simulink model "Two_Zone_MVDC_PSolver_Thermal"  (R2025b)
settings: Solver=FixedStepDiscrete  StartTime=0.0  StopTime=30  FixedStep=TsELEC  RelTol=1e-3  EnableMultiTasking=on
InitFcn:
  | TsELEC = 25e-6;
  | Ts = 25e-6;
  | TsTHERMAL = 1e-3;
  | TsCont = TsELEC;
  | Rsnub = 1e4;
undefined symbols (not defined in the file or in its folder): DiscIntNeverNeededParam, ee_sli_rtmsupport, GABDA, GABDB, GBBDA, GBBDB, gcbh, GPMMA, GPPMB, GPPMC, SADA, SADB, SADC, SADD, SBDA, SBDB, SBDC, SCDA, SCDB, SCDC, SCDD, SDDA, SDDB, SDDC, SDDD, SDDE
libraries: fl_lib x182, nesl_utility x93, ee_lib x50, SimscapeFluids_lib x4, simulink x3, slpidlib x3, eeSmAC1C x2, eePowerMeasurement x2, mcbeeMathTransformLib x2, eeTransforms x1
(part 3 of 5)

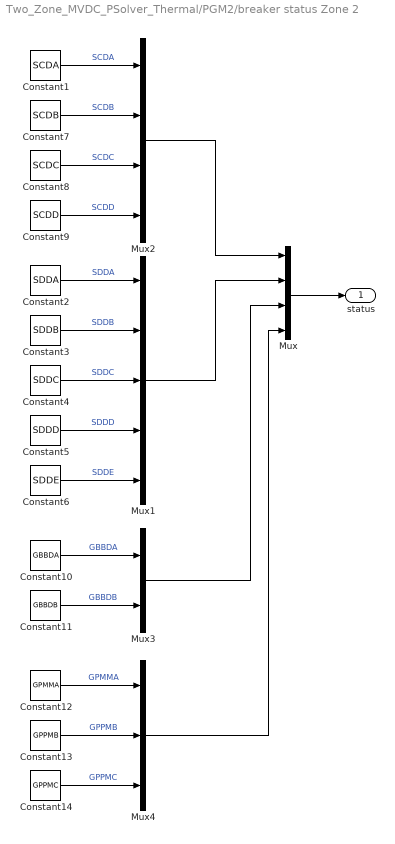
== system Two_Zone_MVDC_PSolver_Thermal/PGM2/breaker status Zone 2 ==
  Constant1 : Constant  Value=SCDA  SampleTime=Ts
  Constant10 : Constant  Value=GBBDA  SampleTime=Ts
  Constant11 : Constant  Value=GBBDB  SampleTime=Ts
  Constant12 : Constant  Value=GPMMA  SampleTime=Ts
  Constant13 : Constant  Value=GPPMB  SampleTime=Ts
  Constant14 : Constant  Value=GPPMC  SampleTime=Ts
  Constant2 : Constant  Value=SDDA  SampleTime=Ts
  Constant3 : Constant  Value=SDDB  SampleTime=Ts
  Constant4 : Constant  Value=SDDC  VectorParams1D=off  SampleTime=Ts
  Constant5 : Constant  Value=SDDD  SampleTime=Ts
  Constant6 : Constant  Value=SDDE  SampleTime=Ts
  Constant7 : Constant  Value=SCDB  SampleTime=Ts
  Constant8 : Constant  Value=SCDC  SampleTime=Ts
  Constant9 : Constant  Value=SCDD  SampleTime=Ts
  Mux : Mux  Inputs=[4 5 2 3]
  Mux1 : Mux  Inputs=5
  Mux2 : Mux
  Mux3 : Mux  Inputs=2
  Mux4 : Mux  Inputs=3
  status : Outport  VectorParamsAs1DForOutWhenUnconnected=off
  wires:
  Mux/1 -> status/1
  Constant9/1 -> Mux2/4  "SCDD"
  Constant8/1 -> Mux2/3  "SCDC"
  Constant7/1 -> Mux2/2  "SCDB"
  Constant1/1 -> Mux2/1  "SCDA"
  Constant6/1 -> Mux1/5  "SDDE"
  Constant4/1 -> Mux1/3  "SDDC"
  Constant3/1 -> Mux1/2  "SDDB"
  Constant2/1 -> Mux1/1  "SDDA"
  Constant5/1 -> Mux1/4  "SDDD"
  Constant10/1 -> Mux3/1  "GBBDA"
  Constant11/1 -> Mux3/2  "GBBDB"
  Constant12/1 -> Mux4/1  "GPMMA"
  Constant13/1 -> Mux4/2  "GPPMB"
  Constant14/1 -> Mux4/3  "GPPMC"
  Mux2/1 -> Mux/1
  Mux1/1 -> Mux/2
  Mux3/1 -> Mux/3
  Mux4/1 -> Mux/4

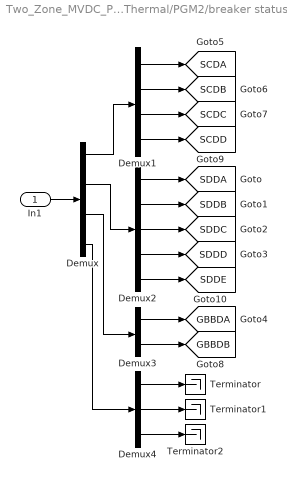
== system Two_Zone_MVDC_PSolver_Thermal/PGM2/breaker status1 ==
  In1 : Inport
  Demux : Demux  Outputs=[4 5 2 3]
  Demux1 : Demux
  Demux2 : Demux  Outputs=5
  Demux3 : Demux  Outputs=2
  Demux4 : Demux  Outputs=3
  Terminator : Terminator
  Terminator1 : Terminator
  Terminator2 : Terminator
  tag scope: GBBDA=global, GBBDB=global, SCDA=global, SCDB=global, SCDC=global, SCDD=global, SDDA=global, SDDB=global, SDDC=global, SDDD=global, SDDE=global
  wires:
  Demux/4 -> Demux4/1
  Demux4/3 -> Terminator2/1
  Demux4/2 -> Terminator1/1
  Demux4/1 -> Terminator/1
  Demux/3 -> Demux3/1
  Demux3/2 -> [GBBDB]
  Demux3/1 -> [GBBDA]
  Demux/2 -> Demux2/1
  Demux/1 -> Demux1/1
  Demux2/5 -> [SDDE]
  Demux1/4 -> [SCDD]
  Demux1/3 -> [SCDC]
  Demux1/2 -> [SCDB]
  Demux1/1 -> [SCDA]
  In1/1 -> Demux/1
  Demux2/4 -> [SDDD]
  Demux2/3 -> [SDDC]
  Demux2/1 -> [SDDA]
  Demux2/2 -> [SDDB]

== system Two_Zone_MVDC_PSolver_Thermal/PMM/Control ==
  Selector : Selector  InputPortWidth=2  IndexOptions=Index vector (dialog)  Indices=2  OutputSizes=1
  Selector1 : Selector  InputPortWidth=2  IndexOptions=Index vector (dialog)  Indices=1  OutputSizes=1
  Speed Control : Subsystem
  Torque Control : Subsystem
  Unit Delay1 : UnitDelay  SampleTime=Ts  HasFrameUpgradeWarning=on
  duty_cycle : Outport
  wires:
  Speed Control/1(IdqRef_PU) -> Torque Control/1(Idq_ref_PU)
  Selector1/1 -> Torque Control/3(Pos_Sim)
  Torque Control/1(Vabc_out_PU) -> Unit Delay1/1
  [Iab_meas1] -> Torque Control/2(Iab_Sim)
  Selector/1 -> Speed Control/2(Speed_Meas_PU)
  [pos_speed_1] -> Selector1/1, Selector/1
  [Nref1] -> Speed Control/1(Speed_Ref_PU)
  Unit Delay1/1 -> duty_cycle/1

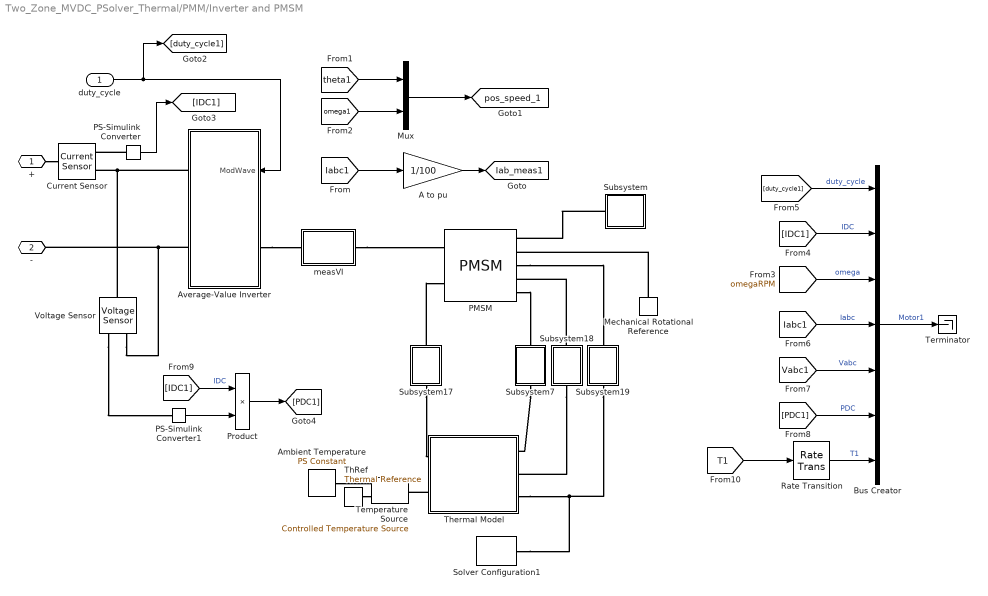
== system Two_Zone_MVDC_PSolver_Thermal/PMM/Inverter and PMSM ==
  duty_cycle : Inport
  A to pu : Gain  Gain=1/100
  Ambient Temperature : fl_lib/Physical Signals/Sources/PS Constant  constant=300
  Average-Value Inverter : Subsystem
  Bus Creator : BusCreator  Inputs=7
  Current Sensor : fl_lib/Electrical/Electrical Sensors/Current Sensor
  Mechanical Rotational Reference : fl_lib/Mechanical/Rotational Elements/Mechanical Rotational Reference
  Mux : Mux  Inputs=2
  PMSM : ee_lib/Electromechanical/Permanent Magnet/PMSM  port_option=ee.enum.threePhasePort.composite  winding_type=ee.enum.statorconnection.wye  machine_param=ee.enum.pmsm.parameterization.constant  nPolePairs=1  pmflux_param=ee.enum.pmflux.fluxlinkage  pm_flux_linkage=3.15*4 Wb  torque_constant=0.18 N*m/A  back_emf_constant=0.18 V/(rad/s)  stator_param=ee.enum.statorparam.LdLqL0  Ld=0.002 H  Lq=0.002 H  idVec=[-200, 0, 200] A  iqVec=[-200, 0, 200] A  LdMatrix=0.0002 * ones(3, 3) H  LqMatrix=0.0002 * ones(3, 3) H  PmMatrix=0.1 * ones(3, 3) Wb  ktMatrix=0.18 * ones(3, 3) N*m/A  keMatrix=0.18 * ones(3, 3) V/(rad/s)  L0=0 H  Ls=0.0002 H  Lm=-0.00002 H  Ms=0.00002 H  Rs=0.01 Ohm  zero_sequence=ee.enum.park.zerosequence.exclude  axes_param=ee.enum.rotorangle.daxis  loss_param=ee.enum.ironloss.none  losses_oc=[0, 0, 0] W  losses_sc=[0, 0, 0] W  f_losses=60 Hz  Isc_losses=95 A  J=2 kg*m^2  lam=1 N*m/(rad/s)  i_d_specify=off  i_d_priority=None  i_d=0 A  i_d_nominal_specify=off  i_d_nominal_value=1  i_d_nominal_unit=A  i_q_specify=off  i_q_priority=None  i_q=0 A  i_q_nominal_specify=off  i_q_nominal_value=1  i_q_nominal_unit=A  torque_specify=off  torque_priority=None  torque=0 N*m  torque_nominal_specify=off  torque_nominal_value=1  torque_nominal_unit=N*m  angular_velocity_specify=off  angular_velocity_priority=High  angular_velocity=0 rpm  angular_velocity_nominal_specify=off  angular_velocity_nominal_value=1  angular_velocity_nominal_unit=rpm  angular_position_specify=off  angular_position_priority=High  angular_position=0 deg  angular_position_nominal_specify=off  angular_position_nominal_value=1  angular_position_nominal_unit=deg  alpha=1e-6 1/K  alpha_flux=-0.001 1/K  Tmeas=298.15 K  stator_thermal_mass=1000 J/K  rotor_thermal_mass=2000 J/K  Rm_percent_rotor=90  Rd_percent_rotor=30  temperatureA_specify=off  temperatureA_priority=High  temperatureA=25 degC  temperatureA_nominal_specify=off  temperatureA_nominal_value=1  temperatureA_nominal_unit=degC  temperatureB_specify=off  temperatureB_priority=High  temperatureB=25 degC  temperatureB_nominal_specify=off  temperatureB_nominal_value=1  temperatureB_nominal_unit=degC  temperatureC_specify=off  temperatureC_priority=High  temperatureC=25 degC  temperatureC_nominal_specify=off  temperatureC_nominal_value=1  temperatureC_nominal_unit=degC  temperatureR_specify=off  temperatureR_priority=High  temperatureR=25 degC  temperatureR_nominal_specify=off  temperatureR_nominal_value=1  temperatureR_nominal_unit=degC
      settings: InternalSimscapePortConfiguration="{\"Bottom\":[],\"Left\":[{\"id\":\"N\",\"label\":\"~\",\"type\":\"foundation.electrical.three_phase\"},{\"id\":\"HR\",\"label\":\"HR\",\"type\":\"foundation.thermal.thermal\"}],\"Right\":[{\"id\":\"R\",\"label\":\"R\",\"type\":\"foundation.mechanical.rotational.rotational\"},{\"id\":\"C\",\"label\":\"C\",\"type\":\"foundation.mechanical.rotational.rotational\"},{\"id\":\"HA\",\"label\":\"HA\",\"type\":\"foundation.thermal.thermal\"},{\"id\":\"HB\",\"label\":\"HB\",\"type\":\"foundation.thermal.thermal\"},{\"id\":\"HC\",\"label\":\"HC\",\"type\":\"foundation.thermal.thermal\"}],\"Top\":[]}"
  PS-Simulink Converter : nesl_utility/PS-Simulink Converter  PhysicalDomain=network_engine_domain  SubClassName=ps_output  LeftPortType=input  RightPortType=output  PseudoPeriodic=off  Frequencies=[]  VectorFormat=1-D array  Unit=inherit  AffineConversion=off
  PS-Simulink Converter1 : nesl_utility/PS-Simulink Converter  PhysicalDomain=network_engine_domain  SubClassName=ps_output  LeftPortType=input  RightPortType=output  PseudoPeriodic=off  Frequencies=[]  VectorFormat=1-D array  Unit=inherit  AffineConversion=off
  Product : Product
  Rate Transition : RateTransition
  Solver Configuration1 : nesl_utility/Solver Configuration  PhysicalDomain=network_engine_domain  SubClassName=solver  LeftPortType=input  RightPortType=generic  Tones=[]  Harmonics=[]  SimulateNoise=off  Profile=off  UseLocalSampling=off  EnableSwitchedLinearOptims=on  FrequencyDomain=off  UseCCode=off  RelTol=0.001  AbsTol=1e-06  MinStep=1e-09  ToWorkspace=off  RevertToSquareIcSolve=off  NumHomotopyIterations=100  PhasorMode=off  PhasorModeNumHarmonics=1  ConsistencySolver=NEWTON_FTOL  IndexReductionMethod=DerivativeReplacement  DoDC=off  ResidualTolerance=1e-9  ConsistencyTolSource=GLOBAL  ConsistencyAbsTol=0.001  ConsistencyRelTol=0.001  ConsistencyTolFactor=0.001  UseLocalSolver=on  LocalSolverChoice=NE_BACKWARD_EULER_ADVANCER  ResolveIndetEquations=on  FunctionEvalNumThread=1  LocalSolverSampleTime=TsTHERMAL  DoFixedCost=on  MaxNonlinIter=1  MaxModeIter=2  ComputeImpulses=off  ImpulseIterations=2  LinearAlgebra=Full  LinearAlgebraNumThread=0  EquationFormulation=NE_TIME_EF  DelaysMemoryBudget=1024  AutomaticFiltering=on  FilteringTimeConstant=0.001  PartitionStorageMethod=AS_NEEDED  PartitionMemoryBudget=1024  PartitionMethod=FAST  MultibodyUseLocalSolver=off  MultibodyLocalSolverChoice=ODE1  MultibodyLocalSolverSampleTime=0.001
  Subsystem : Subsystem
  Subsystem17 : Subsystem
  Subsystem18 : Subsystem
  Subsystem19 : Subsystem
  Subsystem7 : Subsystem
  Temperature Source : fl_lib/Thermal/Thermal Sources/Controlled Temperature Source
  Terminator : Terminator
  ThRef : fl_lib/Thermal/Thermal Elements/Thermal Reference
  Thermal Model : Subsystem  Tag=PublishSubsystem
  Voltage Sensor : fl_lib/Electrical/Electrical Sensors/Voltage Sensor
  measVI : Subsystem
  + : PMIOPort  Side=Left
  - : PMIOPort  Port=2  Side=Left
  tag scope: Iab_meas1=global, pos_speed_1=global
  wires:
  [Vabc1] -> Bus Creator/5  "Vabc"
  [Iabc1] -> Bus Creator/4  "Iabc"
  Bus Creator/1 -> Terminator/1  "Motor1"
  [omegaRPM] -> Bus Creator/3  "omega"
  [IDC1] -> Bus Creator/2  "IDC"
  [duty_cycle1] -> Bus Creator/1  "duty_cycle"
  PS-Simulink Converter/1 -> [IDC1]
  Mux/1 -> [pos_speed_1]
  [omega1] -> Mux/2
  [theta1] -> Mux/1
  [Iabc1] -> A to pu/1
  A to pu/1 -> [Iab_meas1]
  PS-Simulink Converter1/1 -> Product/2
  Product/1 -> [PDC1]
  [PDC1] -> Bus Creator/6  "PDC"
  [IDC1] -> Product/1  "IDC"
  duty_cycle/1 -> [duty_cycle1], Average-Value Inverter/1(ModWave)
  [T1] -> Rate Transition/1
  Rate Transition/1 -> Bus Creator/7  "T1"
  connections:
  Average-Value Inverter/RConn2 -- Voltage Sensor/RConn2 -- -/RConn1
  +/RConn1 -- Current Sensor/LConn1
  PS-Simulink Converter/LConn1 -- Current Sensor/RConn1
  Average-Value Inverter/RConn1 -- Voltage Sensor/LConn1 -- Current Sensor/RConn2
  measVI/RConn1 -- PMSM/LConn1
  Average-Value Inverter/LConn1 -- measVI/LConn1
  Subsystem/RConn1 -- PMSM/RConn1
  Mechanical Rotational Reference/LConn1 -- PMSM/RConn2
  Voltage Sensor/RConn1 -- PS-Simulink Converter1/LConn1
  Subsystem19/LConn1 -- Solver Configuration1/RConn1 -- Thermal Model/RConn3
  Subsystem7/LConn1 -- Thermal Model/RConn1
  Subsystem18/LConn1 -- Thermal Model/RConn2
  Subsystem17/LConn1 -- Thermal Model/LConn1
  ThRef/LConn1 -- Temperature Source/RConn2
  Thermal Model/LConn2 -- Temperature Source/LConn1
  Ambient Temperature/RConn1 -- Temperature Source/RConn1
  Subsystem17/RConn1 -- PMSM/LConn2
  PMSM/RConn3 -- Subsystem19/RConn1
  Subsystem18/RConn1 -- PMSM/RConn4
  PMSM/RConn5 -- Subsystem7/RConn1

== system Two_Zone_MVDC_PSolver_Thermal/PMM/Speed Reference ==
  LPF : Subsystem
  Power Reference : simulink/Sources/Repeating Sequence Interpolated  OutValues=[0 0 0.5 0.5 -0.5 -0.5]  TimeValues=[0 5 10 15 25 100]  LookUpMeth=Interpolation-Use End Values  tsamp=TsELEC  OutMin=[]  OutMax=[]  OutDataTypeStr=double  OutputDataTypeScalingMode=double  OutDataType=fixdt(0,8)  OutScaling=2^-10
  tag scope: Nref1=global
  wires:
  LPF/1(y) -> [Nref1]
  Power Reference/1 -> LPF/1(u)

== system Two_Zone_MVDC_PSolver_Thermal/PGM1/Gas turbine/ AC1C ==
  Constant1 : Constant  Value=0  SampleTime=TsCont
  Constant2 : Constant  Value=0  SampleTime=TsCont
  PS-Simulink Converter : nesl_utility/PS-Simulink Converter  PhysicalDomain=network_engine_domain  SubClassName=ps_output  LeftPortType=input  RightPortType=output  PseudoPeriodic=off  Frequencies=[]  VectorFormat=1-D array  Unit=inherit  AffineConversion=off
  PS-Simulink Converter1 : nesl_utility/PS-Simulink Converter  PhysicalDomain=network_engine_domain  SubClassName=ps_output  LeftPortType=input  RightPortType=output  PseudoPeriodic=off  Frequencies=[]  VectorFormat=1-D array  Unit=inherit  AffineConversion=off
  Rate Transition : RateTransition  OutPortSampleTime=TsELEC
  Rate Transition1 : RateTransition  OutPortSampleTime=TsCont
  Rate Transition2 : RateTransition  OutPortSampleTime=TsCont
  Repeating Sequence Interpolated2 : simulink/Sources/Repeating Sequence Interpolated  OutValues=[1 1 1]  TimeValues=[0 5 1000]  LookUpMeth=Interpolation-Use End Values  tsamp=TsCont  OutMin=[]  OutMax=[]  OutDataTypeStr=double  OutputDataTypeScalingMode=double  OutDataType=fixdt(0,8)  OutScaling=2^-10
  SM AC1C : eeSmAC1C/SM AC1C  E_FD0=1  Ts=TsCont  R_C=0  X_C=0  T_R=0  K_A=80  T_A=0.2  T_B=0  T_C=0  K_F=0.03  T_F=1.49  V_Amax=14.5  V_Amin=-14.5  E_FEmax=6.03  E_FEmin=-5.43  oelInputLocation=Unused  uelInputLocation=Unused  sclInputLocation=Unused  K_E=1  T_E=0.8  K_C=0.2  K_D=0.38  E_1=4.18  S_E_E1=0.1  E_2=3.14  S_E_E2=0.03  V_FEmax=99  V_Emin=0
      settings: LibrarySourceBlock=ee_sl_lib/SM Control/SM AC1C
  Simulink-PS Converter : nesl_utility/Simulink-PS Converter  PhysicalDomain=network_engine_domain  SubClassName=ps_input  LeftPortType=input  RightPortType=output  PseudoPeriodic=off  Frequencies=[]  NoiseDistribution=none  NoiseParameters=[]  Unit=1  AffineConversion=off  FilteringAndDerivatives=provide  SimscapeFilterOrder=1  InputFilterTimeConstant=0.001  UdotUserProvided=0
  Synchronous Machine Field Circuit (pu) : ee_lib/Electromechanical/Synchronous/Synchronous Machine Field Circuit  unit_option=ee.enum.unit.pu  SRated=36e6 V*A  FRated=60 Hz  fieldCircuitParameterization_option=ee.enum.sm.fieldparameterization.current  baseEfd=92.95 V  baseIfd=200 A  parameterization_option=ee.enum.sm.parameterization.standard  Ladu=1.66  Rfd=0.0006  Xl=0.15  Xd=1.81  Xdd=0.3  Xddd=0.23  d_option=ee.enum.circuit.open  Td0d=8 s  Tdd=1.3260 s  Td0dd=0.03 s  Tddd=0.0230 s
      settings: LogSimulationData=on  InternalSimscapePortConfiguration="{\"Bottom\":[],\"Left\":[{\"id\":\"Efd_pu\",\"label\":\"Efd_pu\",\"type\":\"input\"},{\"id\":\"Ifd_pu\",\"label\":\"Ifd_pu\",\"type\":\"output\"}],\"Right\":[{\"id\":\"fd_p\",\"label\":\"fd+\",\"type\":\"foundation.electrical.electrical\"},{\"id\":\"fd_n\",\"label\":\"fd-\",\"type\":\"foundation.electrical.electrical\"}],\"Top\":[]}"
  Terminal Voltage Measurement : ee_lib/Electromechanical/Synchronous/Synchronous Machine Measurement  output_idx=14
      settings: LogSimulationData=on  InternalSimscapePortConfiguration="{\"Bottom\":[],\"Left\":[{\"id\":\"pu_input\",\"label\":\"pu\",\"type\":\"input\"}],\"Right\":[{\"id\":\"pu_output\",\"label\":\"o\",\"type\":\"output\"}],\"Top\":[]}"
  Unit Delay : UnitDelay  InitialCondition=1.37673  SampleTime=-1  HasFrameUpgradeWarning=on
  pu : PMIOPort  Side=Left
  fd+ : PMIOPort  Port=2  Side=Right
  fd- : PMIOPort  Port=3  Side=Right
  wires:
  PS-Simulink Converter1/1 -> Unit Delay/1
  PS-Simulink Converter/1 -> Rate Transition1/1  "Vt1"
  Unit Delay/1 -> Rate Transition2/1  "Ifd1"
  Rate Transition/1 -> Simulink-PS Converter/1
  Repeating Sequence Interpolated2/1 -> SM AC1C/1
  Constant1/1 -> SM AC1C/2
  Rate Transition2/1 -> SM AC1C/10
  Rate Transition1/1 -> SM AC1C/3
  Constant2/1 -> SM AC1C/8, SM AC1C/7, SM AC1C/6, SM AC1C/5, SM AC1C/4, SM AC1C/9
  SM AC1C/1 -> Rate Transition/1
  connections:
  fd-/RConn1 -- Synchronous Machine Field Circuit (pu)/RConn2
  Synchronous Machine Field Circuit (pu)/RConn1 -- fd+/RConn1
  PS-Simulink Converter1/LConn1 -- Synchronous Machine Field Circuit (pu)/LConn2
  Simulink-PS Converter/RConn1 -- Synchronous Machine Field Circuit (pu)/LConn1
  pu/RConn1 -- Terminal Voltage Measurement/LConn1
  PS-Simulink Converter/LConn1 -- Terminal Voltage Measurement/RConn1

== system Two_Zone_MVDC_PSolver_Thermal/PGM1/Gas turbine/Turbine and governor  ==
  Gas Turbine : Subsystem
  Governor : Subsystem
  Ideal Torque Source : fl_lib/Mechanical/Mechanical Sources/Ideal Torque Source
  Mechanical Rotational Reference : fl_lib/Mechanical/Rotational Elements/Mechanical Rotational Reference
  scale by base_torque : fl_lib/Physical Signals/Functions/PS Gain  gain=base_torque N*m/s
  R : PMIOPort  Side=Right
  C : PMIOPort  Port=2  Side=Right
  pu : PMIOPort  Port=3  Side=Left
  connections:
  Gas Turbine/RConn1 -- scale by base_torque/LConn1
  scale by base_torque/RConn1 -- Ideal Torque Source/RConn1
  pu/RConn1 -- Governor/LConn1
  Governor/RConn1 -- Gas Turbine/LConn1
  Ideal Torque Source/LConn1 -- R/RConn1
  Mechanical Rotational Reference/LConn1 -- Ideal Torque Source/RConn2 -- C/RConn1

== system Two_Zone_MVDC_PSolver_Thermal/PGM2/Gas turbine/ AC1C ==
  Constant1 : Constant  Value=0  SampleTime=TsCont
  Constant2 : Constant  Value=0  SampleTime=TsCont
  PS-Simulink Converter : nesl_utility/PS-Simulink Converter  PhysicalDomain=network_engine_domain  SubClassName=ps_output  LeftPortType=input  RightPortType=output  PseudoPeriodic=off  Frequencies=[]  VectorFormat=1-D array  Unit=inherit  AffineConversion=off
  PS-Simulink Converter1 : nesl_utility/PS-Simulink Converter  PhysicalDomain=network_engine_domain  SubClassName=ps_output  LeftPortType=input  RightPortType=output  PseudoPeriodic=off  Frequencies=[]  VectorFormat=1-D array  Unit=inherit  AffineConversion=off
  Rate Transition : RateTransition  OutPortSampleTime=TsELEC
  Rate Transition1 : RateTransition  OutPortSampleTime=TsCont
  Rate Transition2 : RateTransition  OutPortSampleTime=TsCont
  Repeating Sequence Interpolated2 : simulink/Sources/Repeating Sequence Interpolated  OutValues=[1 1 1]  TimeValues=[0 5 1000]  LookUpMeth=Interpolation-Use End Values  tsamp=TsCont  OutMin=[]  OutMax=[]  OutDataTypeStr=double  OutputDataTypeScalingMode=double  OutDataType=fixdt(0,8)  OutScaling=2^-10
  SM AC1C : eeSmAC1C/SM AC1C  E_FD0=1  Ts=TsCont  R_C=0  X_C=0  T_R=0  K_A=80  T_A=0.2  T_B=0  T_C=0  K_F=0.03  T_F=1.49  V_Amax=14.5  V_Amin=-14.5  E_FEmax=6.03  E_FEmin=-5.43  oelInputLocation=Unused  uelInputLocation=Unused  sclInputLocation=Unused  K_E=1  T_E=0.8  K_C=0.2  K_D=0.38  E_1=4.18  S_E_E1=0.1  E_2=3.14  S_E_E2=0.03  V_FEmax=99  V_Emin=0
      settings: LibrarySourceBlock=ee_sl_lib/SM Control/SM AC1C
  Simulink-PS Converter : nesl_utility/Simulink-PS Converter  PhysicalDomain=network_engine_domain  SubClassName=ps_input  LeftPortType=input  RightPortType=output  PseudoPeriodic=off  Frequencies=[]  NoiseDistribution=none  NoiseParameters=[]  Unit=1  AffineConversion=off  FilteringAndDerivatives=provide  SimscapeFilterOrder=1  InputFilterTimeConstant=0.001  UdotUserProvided=0
  Synchronous Machine Field Circuit (pu) : ee_lib/Electromechanical/Synchronous/Synchronous Machine Field Circuit  unit_option=ee.enum.unit.pu  SRated=36e6 V*A  FRated=60 Hz  fieldCircuitParameterization_option=ee.enum.sm.fieldparameterization.current  baseEfd=92.95 V  baseIfd=200 A  parameterization_option=ee.enum.sm.parameterization.standard  Ladu=1.66  Rfd=0.0006  Xl=0.15  Xd=1.81  Xdd=0.3  Xddd=0.23  d_option=ee.enum.circuit.open  Td0d=8 s  Tdd=1.3260 s  Td0dd=0.03 s  Tddd=0.0230 s
      settings: LogSimulationData=on  InternalSimscapePortConfiguration="{\"Bottom\":[],\"Left\":[{\"id\":\"Efd_pu\",\"label\":\"Efd_pu\",\"type\":\"input\"},{\"id\":\"Ifd_pu\",\"label\":\"Ifd_pu\",\"type\":\"output\"}],\"Right\":[{\"id\":\"fd_p\",\"label\":\"fd+\",\"type\":\"foundation.electrical.electrical\"},{\"id\":\"fd_n\",\"label\":\"fd-\",\"type\":\"foundation.electrical.electrical\"}],\"Top\":[]}"
  Terminal Voltage Measurement : ee_lib/Electromechanical/Synchronous/Synchronous Machine Measurement  output_idx=14
      settings: LogSimulationData=on  InternalSimscapePortConfiguration="{\"Bottom\":[],\"Left\":[{\"id\":\"pu_input\",\"label\":\"pu\",\"type\":\"input\"}],\"Right\":[{\"id\":\"pu_output\",\"label\":\"o\",\"type\":\"output\"}],\"Top\":[]}"
  Unit Delay : UnitDelay  InitialCondition=1.37673  SampleTime=-1  HasFrameUpgradeWarning=on
  pu : PMIOPort  Side=Left
  fd+ : PMIOPort  Port=2  Side=Right
  fd- : PMIOPort  Port=3  Side=Right
  wires:
  PS-Simulink Converter1/1 -> Unit Delay/1
  PS-Simulink Converter/1 -> Rate Transition1/1  "Vt2"
  Unit Delay/1 -> Rate Transition2/1  "Ifd2"
  Rate Transition/1 -> Simulink-PS Converter/1
  Repeating Sequence Interpolated2/1 -> SM AC1C/1
  Constant1/1 -> SM AC1C/2
  Rate Transition2/1 -> SM AC1C/10
  Rate Transition1/1 -> SM AC1C/3
  Constant2/1 -> SM AC1C/8, SM AC1C/7, SM AC1C/6, SM AC1C/5, SM AC1C/4, SM AC1C/9
  SM AC1C/1 -> Rate Transition/1
  connections:
  fd-/RConn1 -- Synchronous Machine Field Circuit (pu)/RConn2
  Synchronous Machine Field Circuit (pu)/RConn1 -- fd+/RConn1
  PS-Simulink Converter1/LConn1 -- Synchronous Machine Field Circuit (pu)/LConn2
  Simulink-PS Converter/RConn1 -- Synchronous Machine Field Circuit (pu)/LConn1
  pu/RConn1 -- Terminal Voltage Measurement/LConn1
  PS-Simulink Converter/LConn1 -- Terminal Voltage Measurement/RConn1

== system Two_Zone_MVDC_PSolver_Thermal/PGM2/Gas turbine/Turbine and governor  ==
  Gas Turbine : Subsystem
  Governor : Subsystem
  Ideal Torque Source : fl_lib/Mechanical/Mechanical Sources/Ideal Torque Source
  Mechanical Rotational Reference : fl_lib/Mechanical/Rotational Elements/Mechanical Rotational Reference
  scale by base_torque : fl_lib/Physical Signals/Functions/PS Gain  gain=base_torque N*m/s
  R : PMIOPort  Side=Right
  C : PMIOPort  Port=2  Side=Right
  pu : PMIOPort  Port=3  Side=Left
  connections:
  Gas Turbine/RConn1 -- scale by base_torque/LConn1
  scale by base_torque/RConn1 -- Ideal Torque Source/RConn1
  pu/RConn1 -- Governor/LConn1
  Governor/RConn1 -- Gas Turbine/LConn1
  Ideal Torque Source/LConn1 -- R/RConn1
  Mechanical Rotational Reference/LConn1 -- Ideal Torque Source/RConn2 -- C/RConn1

== system Two_Zone_MVDC_PSolver_Thermal/PMM/Control/Speed Control ==
  Speed_Ref_PU : Inport
  Speed_Meas_PU : Inport  Port=2
  Id_ref : Constant  Value=0  OutDataTypeStr=Inherit: Inherit via back propagation  SampleTime=TsELEC
  Mux1 : Mux  Inputs=2
  PI_Controller_Speed : Subsystem
  IdqRef_PU : Outport  VectorParamsAs1DForOutWhenUnconnected=off
  wires:
  PI_Controller_Speed/1(Iq_ref) -> Mux1/2
  Mux1/1 -> IdqRef_PU/1
  Speed_Meas_PU/1 -> PI_Controller_Speed/2(N_fb)  "speed_meas"
  Speed_Ref_PU/1 -> PI_Controller_Speed/1(N_ref)  "speed_ref"
  Id_ref/1 -> Mux1/1

== system Two_Zone_MVDC_PSolver_Thermal/PMM/Control/Torque Control ==
  Idq_ref_PU : Inport
  Iab_Sim : Inport  Port=2
  Pos_Sim : Inport  Port=3
  Control_System : Subsystem
  Gain : Gain
  Selector : Selector  InputPortWidth=3  IndexOptions=Index vector (dialog)  Indices=[1 2]  OutputSizes=1
  Vabc_out_PU : Outport  InitialOutput=0  VectorParamsAs1DForOutWhenUnconnected=off
  wires:
  Gain/1 -> Control_System/2(Pos_PU)
  Idq_ref_PU/1 -> Control_System/3(Idq_ref_PU)
  Iab_Sim/1 -> Selector/1
  Pos_Sim/1 -> Gain/1
  Control_System/1(Vabc in PU) -> Vabc_out_PU/1
  Selector/1 -> Control_System/1(Iab_meas_PU)

== system Two_Zone_MVDC_PSolver_Thermal/PMM/Inverter and PMSM/Average-Value Inverter ==
  ModWave : Inport
  Average-Value Voltage Source Converter (Three-Phase) : ee_lib/Semiconductors & Converters/Converters/Average-Value Voltage Source Converter (Three-Phase)  port_option=ee.enum.threePhasePort.composite  frequency_option=ee.enum.converters.frequency.variable  input_option=ee.enum.converters.inputOption.ModWave  FRated=60 Hz  losses_parameterization=ee.enum.converters.losses.fixed  Pfixed=1 W  ks=0.01  kc1=1.7 V  kc2=0.01 Ohm  Ploss_vect=[100, 800, 1870, 3250, 4900] W  Irms_vect=[10, 100, 200, 300, 400] A  Vdc_nom=300 V  thermal_mass=30000 J/K  temperature_specify=off  temperature_priority=High  temperature=298.15 K  temperature_nominal_specify=off  temperature_nominal_value=1  temperature_nominal_unit=K
      settings: InternalSimscapePortConfiguration="{\"Bottom\":[],\"Left\":[{\"id\":\"ModWave\",\"label\":\"ModWave\",\"type\":\"input\"},{\"id\":\"N\",\"label\":\"~\",\"type\":\"foundation.electrical.three_phase\"}],\"Right\":[{\"id\":\"p\",\"label\":\"+\",\"type\":\"foundation.electrical.electrical\"},{\"id\":\"n\",\"label\":\"-\",\"type\":\"foundation.electrical.electrical\"}],\"Top\":[]}"
  Simulink-PS Converter : nesl_utility/Simulink-PS Converter  PhysicalDomain=network_engine_domain  SubClassName=ps_input  LeftPortType=input  RightPortType=output  PseudoPeriodic=off  Frequencies=[]  NoiseDistribution=none  NoiseParameters=[]  Unit=1  AffineConversion=off  FilteringAndDerivatives=zero  SimscapeFilterOrder=1  InputFilterTimeConstant=0.001  UdotUserProvided=0
  + : PMIOPort  Side=Right
  ~ : PMIOPort  Port=2  Side=Left
  - : PMIOPort  Port=3  Side=Right
  wires:
  ModWave/1 -> Simulink-PS Converter/1
  connections:
  Average-Value Voltage Source Converter (Three-Phase)/LConn2 -- ~/RConn1
  Average-Value Voltage Source Converter (Three-Phase)/RConn1 -- +/RConn1
  Average-Value Voltage Source Converter (Three-Phase)/RConn2 -- -/RConn1
  Simulink-PS Converter/RConn1 -- Average-Value Voltage Source Converter (Three-Phase)/LConn1

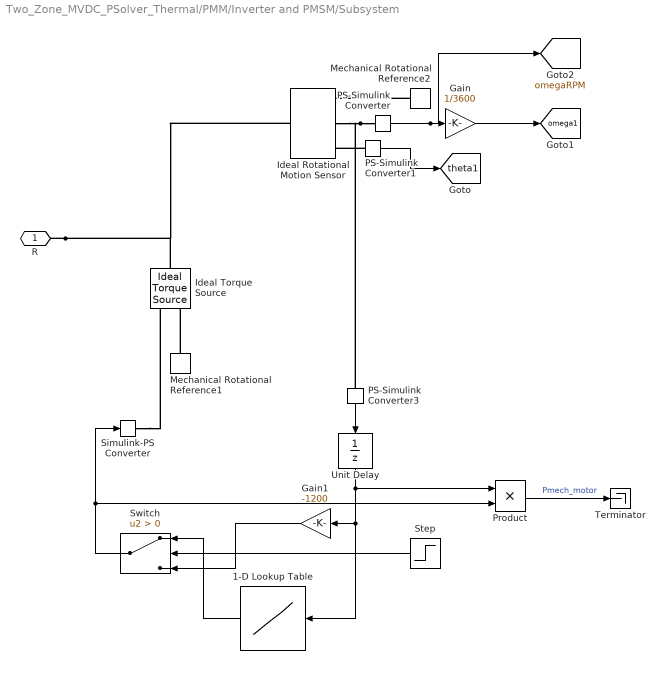
== system Two_Zone_MVDC_PSolver_Thermal/PMM/Inverter and PMSM/Subsystem ==
  1-D Lookup Table : Lookup_n-D  NumberOfTableDimensions=1  BreakpointsForDimension1=[-120*pi 0 50*pi 120*pi]/2  Table=[120*pi*1200 50*pi*1200 0 -120*pi*1200]/2  InternalRulePriority=Speed  RndMeth=Simplest
  Gain : Gain  Gain=1/3600
  Gain1 : Gain  Gain=-1200
  Ideal Rotational Motion Sensor : fl_lib/Mechanical/Mechanical Sensors/Ideal Rotational Motion Sensor  reference=foundation.enum.MeasurementReference.difference  acceleration_port=false  velocity_port=true  position_port=true  wrap_angle=simscape.enum.onoff.off  offset=0 rad
  Ideal Torque Source : fl_lib/Mechanical/Mechanical Sources/Ideal Torque Source
  Mechanical Rotational Reference1 : fl_lib/Mechanical/Rotational Elements/Mechanical Rotational Reference
  Mechanical Rotational Reference2 : fl_lib/Mechanical/Rotational Elements/Mechanical Rotational Reference
  PS-Simulink Converter : nesl_utility/PS-Simulink Converter  PhysicalDomain=network_engine_domain  SubClassName=ps_output  LeftPortType=input  RightPortType=output  PseudoPeriodic=off  Frequencies=[]  VectorFormat=1-D array  Unit=rpm  AffineConversion=off
  PS-Simulink Converter1 : nesl_utility/PS-Simulink Converter  PhysicalDomain=network_engine_domain  SubClassName=ps_output  LeftPortType=input  RightPortType=output  PseudoPeriodic=off  Frequencies=[]  VectorFormat=1-D array  Unit=inherit  AffineConversion=off
  PS-Simulink Converter3 : nesl_utility/PS-Simulink Converter  PhysicalDomain=network_engine_domain  SubClassName=ps_output  LeftPortType=input  RightPortType=output  PseudoPeriodic=off  Frequencies=[]  VectorFormat=1-D array  Unit=rad/s  AffineConversion=off
  Product : Product
  Simulink-PS Converter : nesl_utility/Simulink-PS Converter  PhysicalDomain=network_engine_domain  SubClassName=ps_input  LeftPortType=input  RightPortType=output  PseudoPeriodic=off  Frequencies=[]  NoiseDistribution=none  NoiseParameters=[]  Unit=1  AffineConversion=off  FilteringAndDerivatives=provide  SimscapeFilterOrder=1  InputFilterTimeConstant=0.001  UdotUserProvided=0
  Step : Step  Time=12.5  SampleTime=TsELEC
  Switch : Switch  Criteria=u2 > Threshold  SaturateOnIntegerOverflow=off  InputSameDT=off
  Terminator : Terminator
  Unit Delay : UnitDelay  SampleTime=-1  HasFrameUpgradeWarning=on
  "R " : PMIOPort  Side=Right
  tag scope: omega1=global, omegaRPM=global, theta1=global
  wires:
  Switch/1 -> Product/2, Simulink-PS Converter/1
  PS-Simulink Converter3/1 -> Unit Delay/1
  Gain1/1 -> Switch/3
  Unit Delay/1 -> Product/1, Gain1/1, 1-D Lookup Table/1
  Step/1 -> Switch/2
  1-D Lookup Table/1 -> Switch/1
  PS-Simulink Converter1/1 -> [theta1]
  Gain/1 -> [omega1]
  PS-Simulink Converter/1 -> [omegaRPM], Gain/1
  Product/1 -> Terminator/1  "Pmech_motor"
  connections:
  Simulink-PS Converter/RConn1 -- Ideal Torque Source/RConn1
  Mechanical Rotational Reference1/LConn1 -- Ideal Torque Source/RConn2
  Mechanical Rotational Reference2/LConn1 -- Ideal Rotational Motion Sensor/RConn1
  PS-Simulink Converter1/LConn1 -- Ideal Rotational Motion Sensor/RConn3
  PS-Simulink Converter/LConn1 -- PS-Simulink Converter3/LConn1 -- Ideal Rotational Motion Sensor/RConn2
  "R "/RConn1 -- Ideal Torque Source/LConn1 -- Ideal Rotational Motion Sensor/LConn1

== system Two_Zone_MVDC_PSolver_Thermal/PMM/Inverter and PMSM/Subsystem17 ==
  Controlled Temperature Source : fl_lib/Thermal/Thermal Sources/Controlled Temperature Source
  Controlled Heat Flow Rate Source : fl_lib/Thermal/Thermal Sources/Controlled Heat Flow Rate Source
  Heat Flow Rate Sensor : fl_lib/Thermal/Thermal Sensors/Heat Flow Rate Sensor
  PS-Simulink Converter1 : nesl_utility/PS-Simulink Converter  PhysicalDomain=network_engine_domain  SubClassName=ps_output  LeftPortType=input  RightPortType=output  PseudoPeriodic=off  Frequencies=[]  VectorFormat=1-D array  Unit=inherit  AffineConversion=off
  PS-Simulink Converter2 : nesl_utility/PS-Simulink Converter  PhysicalDomain=network_engine_domain  SubClassName=ps_output  LeftPortType=input  RightPortType=output  PseudoPeriodic=off  Frequencies=[]  VectorFormat=1-D array  Unit=inherit  AffineConversion=off
  Rate Transition : RateTransition  Deterministic=off  OutPortSampleTime=TsELEC
  Rate Transition1 : RateTransition  Deterministic=off  InitialCondition=323.15  OutPortSampleTime=TsTHERMAL
  Simulink-PS Converter : nesl_utility/Simulink-PS Converter  PhysicalDomain=network_engine_domain  SubClassName=ps_input  LeftPortType=input  RightPortType=output  PseudoPeriodic=off  Frequencies=[]  NoiseDistribution=none  NoiseParameters=[]  Unit=W  AffineConversion=off  FilteringAndDerivatives=provide  SimscapeFilterOrder=1  InputFilterTimeConstant=0.001  UdotUserProvided=0
  Simulink-PS Converter1 : nesl_utility/Simulink-PS Converter  PhysicalDomain=network_engine_domain  SubClassName=ps_input  LeftPortType=input  RightPortType=output  PseudoPeriodic=off  Frequencies=[]  NoiseDistribution=none  NoiseParameters=[]  Unit=K  AffineConversion=off  FilteringAndDerivatives=provide  SimscapeFilterOrder=1  InputFilterTimeConstant=0.001  UdotUserProvided=0
  Temperature Sensor : fl_lib/Thermal/Thermal Sensors/Temperature Sensor  temperature_measure=foundation.enum.MeasurementReference.difference
  Thermal Reference : fl_lib/Thermal/Thermal Elements/Thermal Reference
  Thermal Reference1 : fl_lib/Thermal/Thermal Elements/Thermal Reference
  b : PMIOPort  Side=Right
  a : PMIOPort  Port=2  Side=Left
  wires:
  PS-Simulink Converter2/1 -> Rate Transition1/1
  PS-Simulink Converter1/1 -> Rate Transition/1
  Rate Transition/1 -> Simulink-PS Converter/1
  Rate Transition1/1 -> Simulink-PS Converter1/1
  connections:
  Controlled Temperature Source/LConn1 -- Heat Flow Rate Sensor/RConn2
  Controlled Temperature Source/RConn2 -- Thermal Reference/LConn1
  PS-Simulink Converter2/LConn1 -- Temperature Sensor/RConn2
  Heat Flow Rate Sensor/RConn1 -- PS-Simulink Converter1/LConn1
  Simulink-PS Converter/RConn1 -- Controlled Heat Flow Rate Source/RConn1
  Simulink-PS Converter1/RConn1 -- Controlled Temperature Source/RConn1
  Controlled Heat Flow Rate Source/RConn2 -- Temperature Sensor/RConn1 -- Thermal Reference1/LConn1
  Controlled Heat Flow Rate Source/LConn1 -- Temperature Sensor/LConn1 -- b/RConn1
  Heat Flow Rate Sensor/LConn1 -- a/RConn1

== system Two_Zone_MVDC_PSolver_Thermal/PMM/Inverter and PMSM/Subsystem18 ==
  Controlled Temperature Source : fl_lib/Thermal/Thermal Sources/Controlled Temperature Source
  Controlled Heat Flow Rate Source : fl_lib/Thermal/Thermal Sources/Controlled Heat Flow Rate Source
  Heat Flow Rate Sensor : fl_lib/Thermal/Thermal Sensors/Heat Flow Rate Sensor
  PS-Simulink Converter1 : nesl_utility/PS-Simulink Converter  PhysicalDomain=network_engine_domain  SubClassName=ps_output  LeftPortType=input  RightPortType=output  PseudoPeriodic=off  Frequencies=[]  VectorFormat=1-D array  Unit=inherit  AffineConversion=off
  PS-Simulink Converter2 : nesl_utility/PS-Simulink Converter  PhysicalDomain=network_engine_domain  SubClassName=ps_output  LeftPortType=input  RightPortType=output  PseudoPeriodic=off  Frequencies=[]  VectorFormat=1-D array  Unit=inherit  AffineConversion=off
  Rate Transition : RateTransition  Deterministic=off  OutPortSampleTime=TsELEC
  Rate Transition1 : RateTransition  Deterministic=off  InitialCondition=323.15  OutPortSampleTime=TsTHERMAL
  Simulink-PS Converter : nesl_utility/Simulink-PS Converter  PhysicalDomain=network_engine_domain  SubClassName=ps_input  LeftPortType=input  RightPortType=output  PseudoPeriodic=off  Frequencies=[]  NoiseDistribution=none  NoiseParameters=[]  Unit=W  AffineConversion=off  FilteringAndDerivatives=provide  SimscapeFilterOrder=1  InputFilterTimeConstant=0.001  UdotUserProvided=0
  Simulink-PS Converter1 : nesl_utility/Simulink-PS Converter  PhysicalDomain=network_engine_domain  SubClassName=ps_input  LeftPortType=input  RightPortType=output  PseudoPeriodic=off  Frequencies=[]  NoiseDistribution=none  NoiseParameters=[]  Unit=K  AffineConversion=off  FilteringAndDerivatives=provide  SimscapeFilterOrder=1  InputFilterTimeConstant=0.001  UdotUserProvided=0
  Temperature Sensor : fl_lib/Thermal/Thermal Sensors/Temperature Sensor  temperature_measure=foundation.enum.MeasurementReference.difference
  Thermal Reference : fl_lib/Thermal/Thermal Elements/Thermal Reference
  Thermal Reference1 : fl_lib/Thermal/Thermal Elements/Thermal Reference
  b : PMIOPort  Side=Right
  a : PMIOPort  Port=2  Side=Left
  wires:
  PS-Simulink Converter2/1 -> Rate Transition1/1
  PS-Simulink Converter1/1 -> Rate Transition/1
  Rate Transition/1 -> Simulink-PS Converter/1
  Rate Transition1/1 -> Simulink-PS Converter1/1
  connections:
  Controlled Temperature Source/LConn1 -- Heat Flow Rate Sensor/RConn2
  Controlled Temperature Source/RConn2 -- Thermal Reference/LConn1
  PS-Simulink Converter2/LConn1 -- Temperature Sensor/RConn2
  Heat Flow Rate Sensor/RConn1 -- PS-Simulink Converter1/LConn1
  Simulink-PS Converter/RConn1 -- Controlled Heat Flow Rate Source/RConn1
  Simulink-PS Converter1/RConn1 -- Controlled Temperature Source/RConn1
  Controlled Heat Flow Rate Source/RConn2 -- Temperature Sensor/RConn1 -- Thermal Reference1/LConn1
  Controlled Heat Flow Rate Source/LConn1 -- Temperature Sensor/LConn1 -- b/RConn1
  Heat Flow Rate Sensor/LConn1 -- a/RConn1

== system Two_Zone_MVDC_PSolver_Thermal/PMM/Inverter and PMSM/Subsystem19 ==
  Controlled Temperature Source : fl_lib/Thermal/Thermal Sources/Controlled Temperature Source
  Controlled Heat Flow Rate Source : fl_lib/Thermal/Thermal Sources/Controlled Heat Flow Rate Source
  Heat Flow Rate Sensor : fl_lib/Thermal/Thermal Sensors/Heat Flow Rate Sensor
  PS-Simulink Converter1 : nesl_utility/PS-Simulink Converter  PhysicalDomain=network_engine_domain  SubClassName=ps_output  LeftPortType=input  RightPortType=output  PseudoPeriodic=off  Frequencies=[]  VectorFormat=1-D array  Unit=inherit  AffineConversion=off
  PS-Simulink Converter2 : nesl_utility/PS-Simulink Converter  PhysicalDomain=network_engine_domain  SubClassName=ps_output  LeftPortType=input  RightPortType=output  PseudoPeriodic=off  Frequencies=[]  VectorFormat=1-D array  Unit=inherit  AffineConversion=off
  Rate Transition : RateTransition  Deterministic=off  OutPortSampleTime=TsELEC
  Rate Transition1 : RateTransition  Deterministic=off  InitialCondition=323.15  OutPortSampleTime=TsTHERMAL
  Simulink-PS Converter : nesl_utility/Simulink-PS Converter  PhysicalDomain=network_engine_domain  SubClassName=ps_input  LeftPortType=input  RightPortType=output  PseudoPeriodic=off  Frequencies=[]  NoiseDistribution=none  NoiseParameters=[]  Unit=W  AffineConversion=off  FilteringAndDerivatives=provide  SimscapeFilterOrder=1  InputFilterTimeConstant=0.001  UdotUserProvided=0
  Simulink-PS Converter1 : nesl_utility/Simulink-PS Converter  PhysicalDomain=network_engine_domain  SubClassName=ps_input  LeftPortType=input  RightPortType=output  PseudoPeriodic=off  Frequencies=[]  NoiseDistribution=none  NoiseParameters=[]  Unit=K  AffineConversion=off  FilteringAndDerivatives=provide  SimscapeFilterOrder=1  InputFilterTimeConstant=0.001  UdotUserProvided=0
  Temperature Sensor : fl_lib/Thermal/Thermal Sensors/Temperature Sensor  temperature_measure=foundation.enum.MeasurementReference.difference
  Thermal Reference : fl_lib/Thermal/Thermal Elements/Thermal Reference
  Thermal Reference1 : fl_lib/Thermal/Thermal Elements/Thermal Reference
  b : PMIOPort  Side=Right
  a : PMIOPort  Port=2  Side=Left
  wires:
  Rate Transition1/1 -> Simulink-PS Converter1/1
  Rate Transition/1 -> Simulink-PS Converter/1
  PS-Simulink Converter1/1 -> Rate Transition/1
  PS-Simulink Converter2/1 -> Rate Transition1/1
  connections:
  Heat Flow Rate Sensor/LConn1 -- a/RConn1
  b/RConn1 -- Temperature Sensor/LConn1 -- Controlled Heat Flow Rate Source/LConn1
  Thermal Reference1/LConn1 -- Temperature Sensor/RConn1 -- Controlled Heat Flow Rate Source/RConn2
  Simulink-PS Converter1/RConn1 -- Controlled Temperature Source/RConn1
  Simulink-PS Converter/RConn1 -- Controlled Heat Flow Rate Source/RConn1
  Heat Flow Rate Sensor/RConn1 -- PS-Simulink Converter1/LConn1
  PS-Simulink Converter2/LConn1 -- Temperature Sensor/RConn2
  Controlled Temperature Source/RConn2 -- Thermal Reference/LConn1
  Controlled Temperature Source/LConn1 -- Heat Flow Rate Sensor/RConn2

== system Two_Zone_MVDC_PSolver_Thermal/PMM/Inverter and PMSM/Subsystem7 ==
  Controlled Temperature Source : fl_lib/Thermal/Thermal Sources/Controlled Temperature Source
  Controlled Heat Flow Rate Source : fl_lib/Thermal/Thermal Sources/Controlled Heat Flow Rate Source
  Heat Flow Rate Sensor : fl_lib/Thermal/Thermal Sensors/Heat Flow Rate Sensor
  PS-Simulink Converter1 : nesl_utility/PS-Simulink Converter  PhysicalDomain=network_engine_domain  SubClassName=ps_output  LeftPortType=input  RightPortType=output  PseudoPeriodic=off  Frequencies=[]  VectorFormat=1-D array  Unit=inherit  AffineConversion=off
  PS-Simulink Converter2 : nesl_utility/PS-Simulink Converter  PhysicalDomain=network_engine_domain  SubClassName=ps_output  LeftPortType=input  RightPortType=output  PseudoPeriodic=off  Frequencies=[]  VectorFormat=1-D array  Unit=inherit  AffineConversion=off
  Rate Transition : RateTransition  Deterministic=off  OutPortSampleTime=TsELEC
  Rate Transition1 : RateTransition  Deterministic=off  InitialCondition=323.15  OutPortSampleTime=TsTHERMAL
  Simulink-PS Converter : nesl_utility/Simulink-PS Converter  PhysicalDomain=network_engine_domain  SubClassName=ps_input  LeftPortType=input  RightPortType=output  PseudoPeriodic=off  Frequencies=[]  NoiseDistribution=none  NoiseParameters=[]  Unit=W  AffineConversion=off  FilteringAndDerivatives=provide  SimscapeFilterOrder=1  InputFilterTimeConstant=0.001  UdotUserProvided=0
  Simulink-PS Converter1 : nesl_utility/Simulink-PS Converter  PhysicalDomain=network_engine_domain  SubClassName=ps_input  LeftPortType=input  RightPortType=output  PseudoPeriodic=off  Frequencies=[]  NoiseDistribution=none  NoiseParameters=[]  Unit=K  AffineConversion=off  FilteringAndDerivatives=provide  SimscapeFilterOrder=1  InputFilterTimeConstant=0.001  UdotUserProvided=0
  Temperature Sensor : fl_lib/Thermal/Thermal Sensors/Temperature Sensor  temperature_measure=foundation.enum.MeasurementReference.difference
  Thermal Reference : fl_lib/Thermal/Thermal Elements/Thermal Reference
  Thermal Reference1 : fl_lib/Thermal/Thermal Elements/Thermal Reference
  b : PMIOPort  Side=Right
  a : PMIOPort  Port=2  Side=Left
  wires:
  Rate Transition1/1 -> Simulink-PS Converter1/1
  Rate Transition/1 -> Simulink-PS Converter/1
  PS-Simulink Converter1/1 -> Rate Transition/1
  PS-Simulink Converter2/1 -> Rate Transition1/1
  connections:
  Heat Flow Rate Sensor/LConn1 -- a/RConn1
  b/RConn1 -- Temperature Sensor/LConn1 -- Controlled Heat Flow Rate Source/LConn1
  Thermal Reference1/LConn1 -- Temperature Sensor/RConn1 -- Controlled Heat Flow Rate Source/RConn2
  Simulink-PS Converter1/RConn1 -- Controlled Temperature Source/RConn1
  Simulink-PS Converter/RConn1 -- Controlled Heat Flow Rate Source/RConn1
  Heat Flow Rate Sensor/RConn1 -- PS-Simulink Converter1/LConn1
  PS-Simulink Converter2/LConn1 -- Temperature Sensor/RConn2
  Controlled Temperature Source/RConn2 -- Thermal Reference/LConn1
  Controlled Temperature Source/LConn1 -- Heat Flow Rate Sensor/RConn2
